simulink model "tether_dynamics"  (R2023a)
settings: Solver=ode5  StartTime=0.0  StopTime=30  FixedStep=0.0001  RelTol=1e-2
undefined symbols (not defined in the file): ext, ics, P0, P1, P10, P2, P3, P4, P5, P6, P7, P8, P9
settings Model: Creator=Dizzy  LastModifiedBy=dmmavani
settings OptimizationCC: DefaultParameterBehavior=Inlined  EnhancedBackFolding=on  PassReuseOutputArgsAs=Individual arguments  ZeroExternalMemoryAtStartup=off  ZeroInternalMemoryAtStartup=off  OptimizeBlockOrder=speed  DifferentSizesBufferReuse=on  OptimizationCustomize=off  EfficientTunableParamExpr=on
settings DebuggingCC: ParameterTunabilityLossMsg=error
settings SFSimCC: MATLABDynamicMemAlloc=off
settings RTWCC: Description=Embedded Coder  SystemTargetFile=ert.tlc  TemplateMakefile=ert_default_tmf
settings CodeAppCC: ForceParamTrailComments=on  IgnoreCustomStorageClasses=off  OperatorAnnotations=on  SimulinkDataObjDesc=on  SFDataObjDesc=on  InsertBlockDesc=on
settings ERTTargetCC: TargetLangStandard=C99 (ISO)  GenerateSampleERTMain=on  InlinedParameterPlacement=NonHierarchical  ERTCustomFileTemplate=example_file_process.tlc

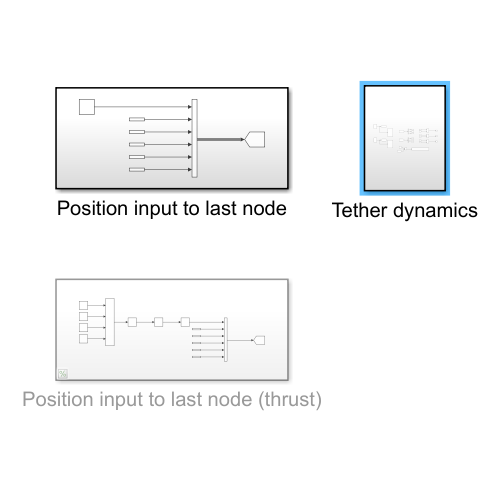
[thumbnail: Simulink's stored preview of the top-level diagram]
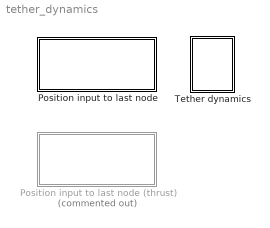
== system tether_dynamics ==
  Position input to last node : Subsystem
  Position input to last node (thrust) : Subsystem  Commented=on
  Tether dynamics : Subsystem

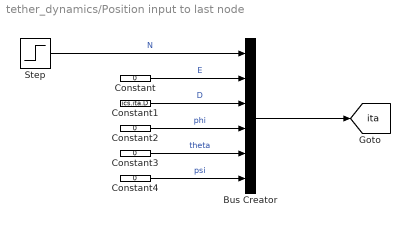
== system tether_dynamics/Position input to last node ==
  Bus Creator : BusCreator  Inputs=6  OutDataTypeStr=Bus: ita
  Constant{,2..4} (4 alike) : Constant  Value=0
  Constant1 : Constant  Value=ics.ita.D
  Step : Step  Time=0  SampleTime=0
  tag scope: ita=global
  wires:
  Constant1/1 -> Bus Creator/3  "D"
  Constant3/1 -> Bus Creator/5  "theta"
  Constant/1 -> Bus Creator/2  "E"
  Bus Creator/1 -> [ita]
  Constant2/1 -> Bus Creator/4  "phi"
  Constant4/1 -> Bus Creator/6  "psi"
  Step/1 -> Bus Creator/1  "N"

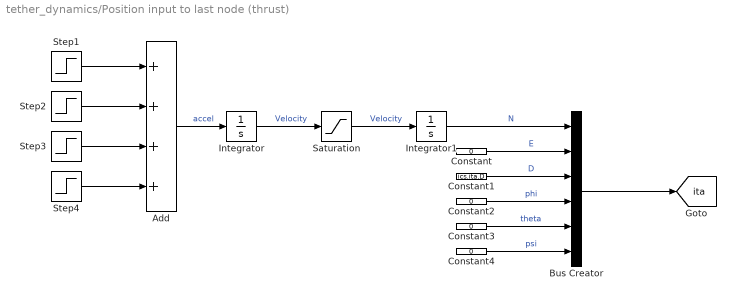
== system tether_dynamics/Position input to last node (thrust) ==
  Add : Sum  Inputs=++++
  Bus Creator : BusCreator  Inputs=6  OutDataTypeStr=Bus: ita
  Constant{,2..4} (4 alike) : Constant  Value=0
  Constant1 : Constant  Value=ics.ita.D
  Integrator : Integrator
  Integrator1 : Integrator
  Saturation : Saturate  UpperLimit=0.7  LowerLimit=0
  Step1 : Step  After=0.1  SampleTime=0
  Step2 : Step  Time=5  Before=0.1  After=0  SampleTime=0
  Step3 : Step  Time=10  After=-0.1  SampleTime=0
  Step4 : Step  Time=14  Before=-0.1  After=0  SampleTime=0
  tag scope: ita=global
  wires:
  Constant4/1 -> Bus Creator/6  "psi"
  Constant2/1 -> Bus Creator/4  "phi"
  Bus Creator/1 -> [ita]
  Constant/1 -> Bus Creator/2  "E"
  Constant3/1 -> Bus Creator/5  "theta"
  Constant1/1 -> Bus Creator/3  "D"
  Step2/1 -> Add/2
  Add/1 -> Integrator/1  "accel"
  Step1/1 -> Add/1
  Step3/1 -> Add/3
  Step4/1 -> Add/4
  Integrator/1 -> Saturation/1  "Velocity"
  Integrator1/1 -> Bus Creator/1  "N"
  Saturation/1 -> Integrator1/1  "Velocity"

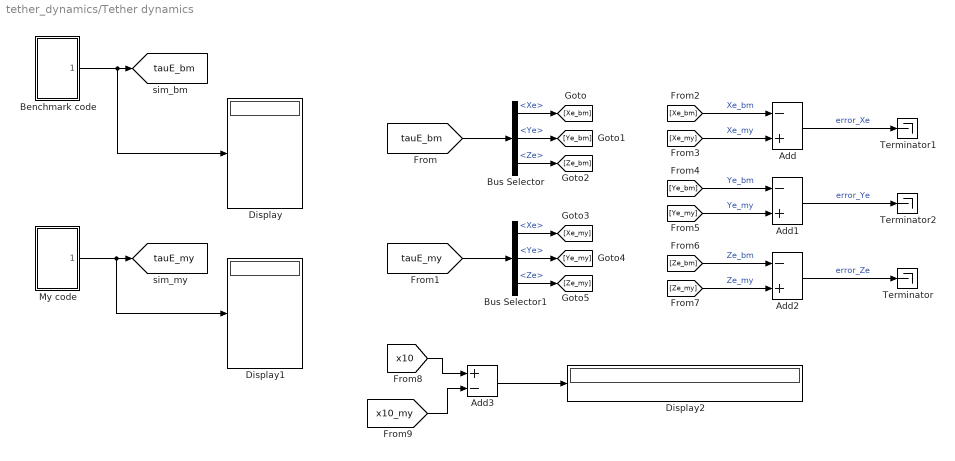
== system tether_dynamics/Tether dynamics ==
  Add : Sum  Inputs=-+
  Add1 : Sum  Inputs=-+
  Add2 : Sum  Inputs=-+
  Add3 : Sum  Inputs=+-
  Benchmark code : Subsystem
  Bus Selector : BusSelector  OutputSignals=Xe,Ye,Ze
  Bus Selector1 : BusSelector  OutputSignals=Xe,Ye,Ze
  Display : Display
  Display1 : Display
  Display2 : Display
  My code : Subsystem
  Terminator : Terminator
  Terminator1 : Terminator
  Terminator2 : Terminator
  tag scope: tauE_bm=global, tauE_my=global
  wires:
  Benchmark code/1(tauExt) -> Display/1, [tauE_bm]
  My code/1(tauExt) -> Display1/1, [tauE_my]
  [Xe_bm] -> Add/1  "Xe_bm"
  Bus Selector1/3 -> [Ze_my]  "<Ze>"
  Bus Selector/3 -> [Ze_bm]  "<Ze>"
  [tauE_my] -> Bus Selector1/1
  Bus Selector1/1 -> [Xe_my]  "<Xe>"
  [Xe_my] -> Add/2  "Xe_my"
  Add2/1 -> Terminator/1  "error_Ze"
  [Ye_bm] -> Add1/1  "Ye_bm"
  Add/1 -> Terminator1/1  "error_Xe"
  [Ze_bm] -> Add2/1  "Ze_bm"
  Bus Selector/1 -> [Xe_bm]  "<Xe>"
  [Ze_my] -> Add2/2  "Ze_my"
  Bus Selector1/2 -> [Ye_my]  "<Ye>"
  Bus Selector/2 -> [Ye_bm]  "<Ye>"
  [Ye_my] -> Add1/2  "Ye_my"
  [tauE_bm] -> Bus Selector/1
  Add1/1 -> Terminator2/1  "error_Ye"
  [x10] -> Add3/1
  [x10_my] -> Add3/2
  Add3/1 -> Display2/1

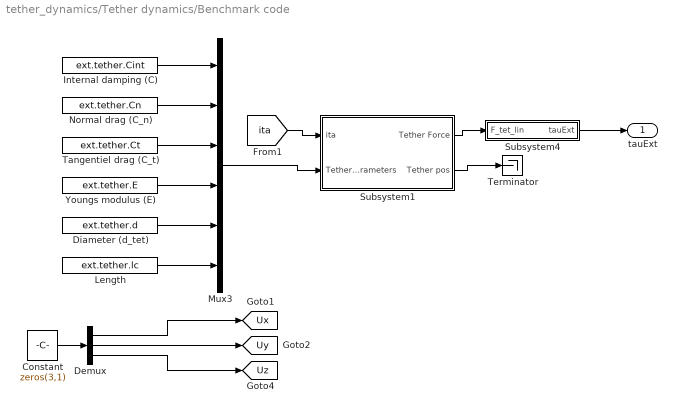
== system tether_dynamics/Tether dynamics/Benchmark code ==
  Constant : Constant  Value=zeros(3,1)
  Demux : Demux  Outputs=3
  Diameter (d_tet) : Constant  Value=ext.tether.d
  Internal damping (C) : Constant  Value=ext.tether.Cint
  Length : Constant  Value=ext.tether.lc
  Mux3 : Mux  Inputs=6
  Normal drag (C_n) : Constant  Value=ext.tether.Cn
  Subsystem1 : Subsystem
  Subsystem4 : Subsystem
  Tangentiel drag (C_t) : Constant  Value=ext.tether.Ct
  Terminator : Terminator
  Youngs modulus (E) : Constant  Value=ext.tether.E
  tauExt : Outport  OutDataTypeStr=Bus: tauExt
  tag scope: Ux=global, Uy=global, Uz=global
  wires:
  [ita] -> Subsystem1/1(ita)
  Demux/2 -> [Uy]
  Subsystem1/1(Tether Force) -> Subsystem4/1(F_tet_lin)
  Demux/3 -> [Uz]
  Constant/1 -> Demux/1
  Normal drag (C_n)/1 -> Mux3/2
  Subsystem1/2(Tether pos) -> Terminator/1
  Length/1 -> Mux3/6
  Subsystem4/1(tauExt) -> tauExt/1
  Demux/1 -> [Ux]
  Internal damping (C)/1 -> Mux3/1
  Tangentiel drag (C_t)/1 -> Mux3/3
  Diameter (d_tet)/1 -> Mux3/5
  Youngs modulus (E)/1 -> Mux3/4
  Mux3/1 -> Subsystem1/2(Tether_Parameters)

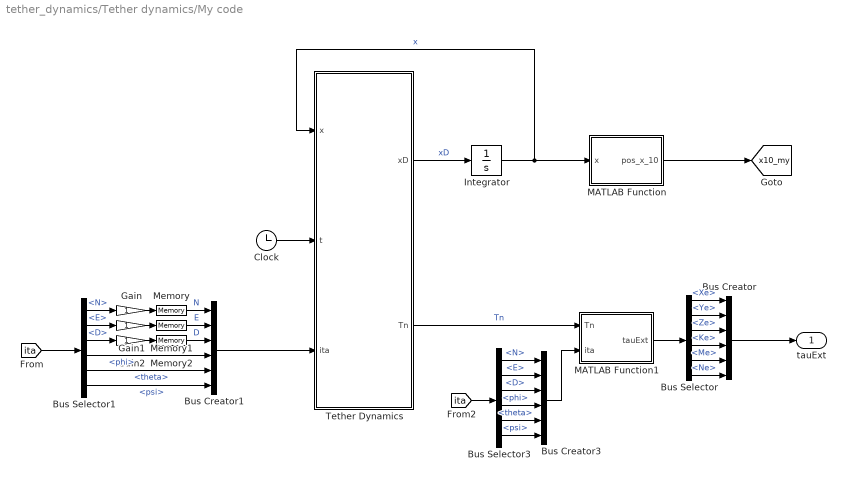
== system tether_dynamics/Tether dynamics/My code ==
  Bus Creator : BusCreator  Inputs=6  OutDataTypeStr=Bus: tauExt
  Bus Creator1 : BusCreator  Inputs=6  OutDataTypeStr=Bus: ita
  Bus Creator3 : BusCreator  Inputs=6  OutDataTypeStr=Bus: ita
  Bus Selector : BusSelector  OutputSignals=Xe,Ye,Ze,Ke,Me,Ne
  Bus Selector1 : BusSelector  OutputSignals=N,E,D,phi,theta,psi
  Bus Selector3 : BusSelector  OutputSignals=N,E,D,phi,theta,psi
  Clock : Clock
  Gain : Gain
  Gain1 : Gain
  Gain2 : Gain
  Integrator : Integrator  InitialCondition=ics.tether.xstate
  MATLAB Function : MATLAB Function  TreatAsAtomicUnit=on
  MATLAB Function1 : MATLAB Function  TreatAsAtomicUnit=on
  Memory : Memory  InitialCondition=ics.ita.N
  Memory1 : Memory  InitialCondition=ics.ita.E
  Memory2 : Memory  InitialCondition=ics.ita.D
  Tether Dynamics : MATLAB Function  TreatAsAtomicUnit=on
  tauExt : Outport  OutDataTypeStr=Bus: tauExt
  tag scope: x10_my=global
  wires:
  Bus Creator1/1 -> Tether Dynamics/3(ita)
  Bus Selector1/4 -> Bus Creator1/4  "<phi>"
  Tether Dynamics/1(xD) -> Integrator/1  "xD"
  Bus Selector3/5 -> Bus Creator3/5  "<theta>"
  Bus Selector/3 -> Bus Creator/3  "<Ze>"
  Bus Selector3/3 -> Bus Creator3/3  "<D>"
  Bus Selector1/2 -> Gain1/1  "<E>"
  Integrator/1 -> Tether Dynamics/1(x), MATLAB Function/1(x)  "x"
  Memory2/1 -> Bus Creator1/3  "D"
  Bus Selector/5 -> Bus Creator/5  "<Me>"
  Bus Creator3/1 -> MATLAB Function1/2(ita)
  Bus Selector/4 -> Bus Creator/4  "<Ke>"
  Bus Selector1/1 -> Gain/1  "<N>"
  Gain/1 -> Memory/1
  Memory/1 -> Bus Creator1/1  "N"
  Bus Selector3/6 -> Bus Creator3/6  "<psi>"
  MATLAB Function1/1(tauExt) -> Bus Selector/1
  Bus Selector3/1 -> Bus Creator3/1  "<N>"
  Bus Selector/2 -> Bus Creator/2  "<Ye>"
  Bus Selector3/2 -> Bus Creator3/2  "<E>"
  Bus Selector/6 -> Bus Creator/6  "<Ne>"
  Bus Selector3/4 -> Bus Creator3/4  "<phi>"
  Bus Selector1/3 -> Gain2/1  "<D>"
  Bus Selector/1 -> Bus Creator/1  "<Xe>"
  Tether Dynamics/2(Tn) -> MATLAB Function1/1(Tn)  "Tn"
  [ita] -> Bus Selector3/1
  Clock/1 -> Tether Dynamics/2(t)
  Bus Selector1/5 -> Bus Creator1/5  "<theta>"
  [ita] -> Bus Selector1/1
  Bus Creator/1 -> tauExt/1
  Bus Selector1/6 -> Bus Creator1/6  "<psi>"
  Gain2/1 -> Memory2/1
  Gain1/1 -> Memory1/1
  Memory1/1 -> Bus Creator1/2  "E"
  MATLAB Function/1(pos_x_10) -> [x10_my]

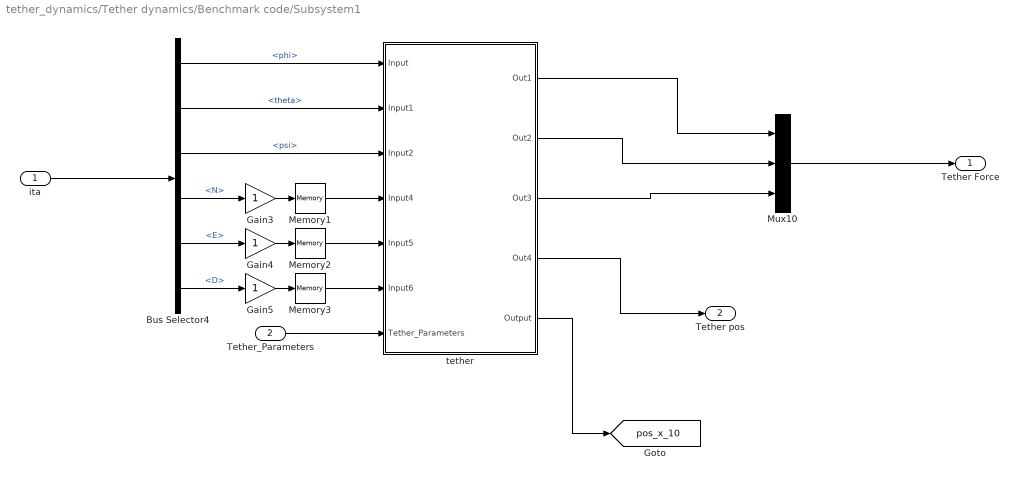
== system tether_dynamics/Tether dynamics/Benchmark code/Subsystem1 ==
  ita : Inport  OutDataTypeStr=Bus: ita
  Tether_Parameters : Inport  Port=2
  Bus Selector4 : BusSelector  OutputSignals=phi,theta,psi,N,E,D
  Gain3 : Gain
  Gain4 : Gain
  Gain5 : Gain
  Memory1 : Memory  InitialCondition=P10(1)
  Memory2 : Memory  InitialCondition=P10(2)
  Memory3 : Memory  InitialCondition=P10(3)
  Mux10 : Mux  Inputs=3
  tether : Subsystem
  Tether Force : Outport
  Tether pos : Outport  Port=2
  tag scope: pos_x_10=global
  wires:
  Memory3/1 -> tether/6(Input6)
  Memory2/1 -> tether/5(Input5)
  Memory1/1 -> tether/4(Input4)
  Bus Selector4/1 -> tether/1(Input)  "<phi>"
  Bus Selector4/2 -> tether/2(Input1)  "<theta>"
  Bus Selector4/3 -> tether/3(Input2)  "<psi>"
  Tether_Parameters/1 -> tether/7(Tether_Parameters)
  Gain3/1 -> Memory1/1
  Gain4/1 -> Memory2/1
  Gain5/1 -> Memory3/1
  tether/1(Out1) -> Mux10/1
  tether/2(Out2) -> Mux10/2
  tether/3(Out3) -> Mux10/3
  Mux10/1 -> Tether Force/1
  tether/4(Out4) -> Tether pos/1
  Bus Selector4/4 -> Gain3/1  "<N>"
  Bus Selector4/5 -> Gain4/1  "<E>"
  Bus Selector4/6 -> Gain5/1  "<D>"
  ita/1 -> Bus Selector4/1
  tether/5(Output) -> [pos_x_10]

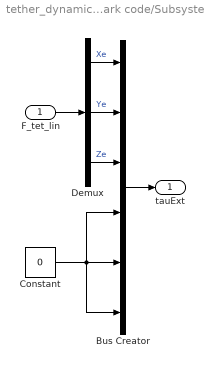
== system tether_dynamics/Tether dynamics/Benchmark code/Subsystem4 ==
  F_tet_lin : Inport
  Bus Creator : BusCreator  Inputs=6  OutDataTypeStr=Bus: tauExt
      settings: InheritFromInputs=off
  Constant : Constant  Value=0
  Demux : Demux  Outputs=3
  tauExt : Outport  OutDataTypeStr=Bus: tauExt
  wires:
  Constant/1 -> Bus Creator/6, Bus Creator/4, Bus Creator/5
  Bus Creator/1 -> tauExt/1
  Demux/1 -> Bus Creator/1  "Xe"
  Demux/2 -> Bus Creator/2  "Ye"
  Demux/3 -> Bus Creator/3  "Ze"
  F_tet_lin/1 -> Demux/1

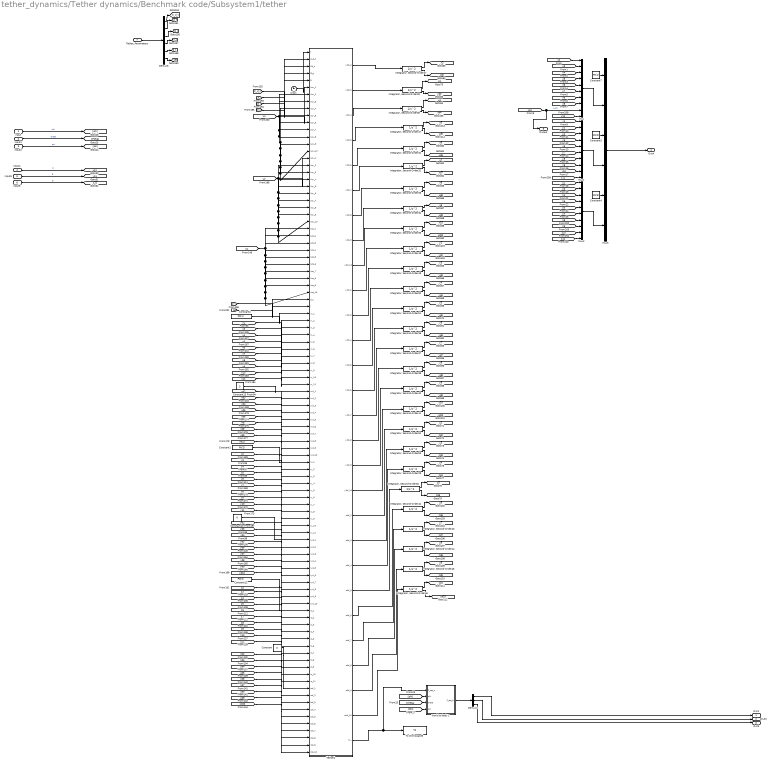
== system tether_dynamics/Tether dynamics/Benchmark code/Subsystem1/tether ==
  Input : Inport
  Input1 : Inport  Port=2
  Input2 : Inport  Port=3
  Input4 : Inport  Port=4
  Input5 : Inport  Port=5
  Input6 : Inport  Port=6
  Tether_Parameters : Inport  Port=7
  Clock : Clock
  Constant : Constant  Value=0
  Constant1 : Constant  Value=P0(2)
  Constant10 : Constant  Value=0
  Constant12 : Constant  Value=P0(3)
  Constant13 : Constant  Value=0
  Constant2 : Constant  Value=P0(1)
  Constant3 : Constant  Value=P0(2)
  Constant4 : Constant  Value=P0(3)
  Constant7 : Constant  Value=P0(1)
  Demux4 : Demux  Outputs=3
  Demux6 : Demux  Outputs=6
  "Integrator, Second-Order27" : SecondOrderIntegrator  ICX=P1(1)
  "Integrator, Second-Order28" : SecondOrderIntegrator  ICX=P2(1)
  "Integrator, Second-Order29" : SecondOrderIntegrator  ICX=P3(3)
  "Integrator, Second-Order30" : SecondOrderIntegrator  ICX=P4(3)
  "Integrator, Second-Order31" : SecondOrderIntegrator  ICX=P5(1)
  "Integrator, Second-Order32" : SecondOrderIntegrator  ICX=P6(1)
  "Integrator, Second-Order33" : SecondOrderIntegrator  ICX=P7(1)
  "Integrator, Second-Order34" : SecondOrderIntegrator  ICX=P8(1)  UpperLimitX=100  LowerLimitX=-100  UpperLimitDXDT=10  LowerLimitDXDT=-10
  "Integrator, Second-Order35" : SecondOrderIntegrator  ICX=P9(1)
  "Integrator, Second-Order36" : SecondOrderIntegrator  ICX=P5(2)
  "Integrator, Second-Order37" : SecondOrderIntegrator  ICX=P6(2)
  "Integrator, Second-Order38" : SecondOrderIntegrator  ICX=P7(2)
  "Integrator, Second-Order39" : SecondOrderIntegrator  ICX=P3(1)
  "Integrator, Second-Order40" : SecondOrderIntegrator  ICX=P8(2)
  "Integrator, Second-Order41" : SecondOrderIntegrator  ICX=P9(2)
  "Integrator, Second-Order42" : SecondOrderIntegrator  ICX=P5(3)
  "Integrator, Second-Order43" : SecondOrderIntegrator  ICX=P6(3)
  "Integrator, Second-Order44" : SecondOrderIntegrator  ICX=P7(3)
  "Integrator, Second-Order45" : SecondOrderIntegrator  ICX=P8(3)
  "Integrator, Second-Order46" : SecondOrderIntegrator  ICX=P9(3)
  "Integrator, Second-Order47" : SecondOrderIntegrator  ICX=P4(1)
  "Integrator, Second-Order48" : SecondOrderIntegrator  ICX=P1(2)
  "Integrator, Second-Order49" : SecondOrderIntegrator  ICX=P2(2)
  "Integrator, Second-Order50" : SecondOrderIntegrator  ICX=P3(2)
  "Integrator, Second-Order51" : SecondOrderIntegrator  ICX=P4(2)
  "Integrator, Second-Order52" : SecondOrderIntegrator  ICX=P1(3)
  "Integrator, Second-Order53" : SecondOrderIntegrator  ICX=P2(3)
  Mux : Mux  Inputs=10
  Mux1 : Mux  Inputs=10
  Mux2 : Mux  Inputs=10
  Mux3 : Mux  Inputs=6
  Tether2 : MATLAB Function  TreatAsAtomicUnit=on
  To Workspace3 : ToWorkspace  VariableName=T2  SaveFormat=Timeseries  SampleTime=-1
  World to body 1 : MATLAB Function  TreatAsAtomicUnit=on
  Out1 : Outport
  Out2 : Outport  Port=2
  Out3 : Outport  Port=3
  Out4 : Outport  Port=4
  Output : Outport  Port=5
  tag scope: C_d_t=global, Cd_t=global, Ct_t=global, Em_t=global, I_tet=global, d_t=global, x10=global, x11=global, x2=global, x3=global, x4=global, x5=global, x6=global, x7=global, x8=global, x9=global, xd10=global, xd2=global, xd3=global, xd4=global, xd5=global, xd6=global, xd7=global, xd8=global, xd9=global, y10=global, y11=global, y2=global, y3=global, y4=global, y5=global, y6=global, y7=global, y8=global, y9=global, yd10=global, yd2=global, yd3=global, yd4=global, yd5=global, yd6=global, yd7=global, yd8=global, yd9=global, z10=global, z11=global, z2=global, z3=global, z4=global, z5=global, z6=global, z7=global, z8=global, z9=global, zd10=global, zd2=global, zd3=global, zd4=global, zd5=global, zd6=global, zd7=global, zd8=global, zd9=global
  wires:
  Input/1 -> [phi]  "phi"
  Input1/1 -> [theta]  "theta"
  Input2/1 -> [psi]  "psi"
  Input4/1 -> [x11]  "N"
  Input5/1 -> [y11]  "E"
  Input6/1 -> [z11]  "D"
  "Integrator, Second-Order46"/1 -> [z10]
  "Integrator, Second-Order52"/1 -> [z2]
  [zd7] -> Tether2/97(rzd_7)
  "Integrator, Second-Order28"/2 -> [xd3]
  "Integrator, Second-Order36"/1 -> [y6]
  "Integrator, Second-Order32"/1 -> [x7]
  [yd7] -> Tether2/76(ryd_7)
  [zd3] -> Tether2/93(rzd_3)
  Constant12/1 -> Tether2/80(rz_1)
  "Integrator, Second-Order29"/2 -> [zd4]
  "Integrator, Second-Order29"/1 -> [z4]
  "Integrator, Second-Order35"/2 -> [xd10]
  [y5] -> Tether2/63(ry_5)
  "Integrator, Second-Order52"/2 -> [zd2]
  [z8] -> Tether2/87(rz_8)
  "Integrator, Second-Order50"/1 -> [y4]
  [y6] -> Tether2/64(ry_6)
  [xd5] -> Tether2/53(rxd_5)
  "Integrator, Second-Order50"/2 -> [yd4]
  "Integrator, Second-Order53"/1 -> [z3]
  [zd5] -> Tether2/95(rzd_5)
  [zd10] -> Tether2/100(rzd_10)
  [xd9] -> Tether2/57(rxd_9)
  [zd6] -> Tether2/96(rzd_6)
  [yd3] -> Tether2/72(ryd_3)
  "Integrator, Second-Order41"/2 -> [yd10]
  [z9] -> Tether2/88(rz_9)
  "Integrator, Second-Order38"/1 -> [y8]
  "Integrator, Second-Order31"/2 -> [xd6]
  "Integrator, Second-Order33"/2 -> [xd8]
  [yd8] -> Tether2/77(ryd_8)
  "Integrator, Second-Order41"/1 -> [y10]
  "Integrator, Second-Order30"/1 -> [z5]
  Constant1/1 -> Tether2/59(ry_1)
  [y9] -> Tether2/67(ry_9)
  "Integrator, Second-Order46"/2 -> [zd10]
  [yd10] -> Tether2/79(ryd_10)
  [z4] -> Tether2/83(rz_4)
  [y10] -> Tether2/68(ry_10)
  "Integrator, Second-Order48"/1 -> [y2]
  "Integrator, Second-Order45"/2 -> [zd9]
  [zd4] -> Tether2/94(rzd_4)
  [z11] -> Tether2/90(rz_11)
  "Integrator, Second-Order47"/2 -> [xd5]
  [y4] -> Tether2/62(ry_4)
  "Integrator, Second-Order31"/1 -> [x6]
  [z3] -> Tether2/82(rz_3)
  [xd4] -> Tether2/52(rxd_4)
  "Integrator, Second-Order37"/2 -> [yd7]
  [x7] -> Tether2/44(rx_7)
  [zd9] -> Tether2/99(rzd_9)
  [x3] -> Tether2/40(rx_3)
  [yd5] -> Tether2/74(ryd_5)
  "Integrator, Second-Order44"/2 -> [zd8]
  "Integrator, Second-Order40"/1 -> [y9]
  "Integrator, Second-Order27"/1 -> [x2]
  "Integrator, Second-Order48"/2 -> [yd2]
  [yd2] -> Tether2/71(ryd_2)
  "Integrator, Second-Order51"/2 -> [yd5]
  "Integrator, Second-Order36"/2 -> [yd6]
  "Integrator, Second-Order47"/1 -> [x5]
  "Integrator, Second-Order49"/1 -> [y3]
  "Integrator, Second-Order32"/2 -> [xd7]
  [x4] -> Tether2/41(rx_4)
  "Integrator, Second-Order45"/1 -> [z9]
  [xd8] -> Tether2/56(rxd_8)
  "Integrator, Second-Order37"/1 -> [y7]
  [z6] -> Tether2/85(rz_6)
  "Integrator, Second-Order40"/2 -> [yd9]
  "Integrator, Second-Order43"/1 -> [z7]
  "Integrator, Second-Order51"/1 -> [y5]
  Constant2/1 -> Tether2/38(rx_1)
  "Integrator, Second-Order34"/1 -> [x9]
  "Integrator, Second-Order44"/1 -> [z8]
  "Integrator, Second-Order28"/1 -> [x3]
  [z5] -> Tether2/84(rz_5)
  "Integrator, Second-Order39"/1 -> [x4]
  [z7] -> Tether2/86(rz_7)
  [z2] -> Tether2/81(rz_2)
  [xd6] -> Tether2/54(rxd_6)
  "Integrator, Second-Order34"/2 -> [xd9]
  [yd4] -> Tether2/73(ryd_4)
  [x6] -> Tether2/43(rx_6)
  [zd8] -> Tether2/98(rzd_8)
  [x8] -> Tether2/45(rx_8)
  [xd10] -> Tether2/58(rxd_10)
  [x5] -> Tether2/42(rx_5)
  [y7] -> Tether2/65(ry_7)
  [yd6] -> Tether2/75(ryd_6)
  [zd2] -> Tether2/92(rzd_2)
  "Integrator, Second-Order35"/1 -> [x10]
  [xd3] -> Tether2/51(rxd_3)
  "Integrator, Second-Order30"/2 -> [zd5]
  [y2] -> Tether2/60(ry_2)
  "Integrator, Second-Order49"/2 -> [yd3]
  "Integrator, Second-Order27"/2 -> [xd2]
  [y11] -> Tether2/69(ry_11)
  [xd7] -> Tether2/55(rxd_7)
  [yd9] -> Tether2/78(ryd_9)
  [y8] -> Tether2/66(ry_8)
  [z10] -> Tether2/89(rz_10)
  "Integrator, Second-Order42"/2 -> [zd6]
  [x10] -> Tether2/47(rx_10)
  [x2] -> Tether2/39(rx_2)
  [Uz] -> Tether2/35(Ucz_10), Tether2/34(Ucz_9), Tether2/33(Ucz_8), Tether2/32(Ucz_7), Tether2/31(Ucz_6), Tether2/30(Ucz_5), Tether2/29(Ucz_4), Tether2/28(Ucz_3), Tether2/27(Ucz_2), Tether2/26(Ucz_1)
  [x11] -> Tether2/48(rx_11)
  "Integrator, Second-Order33"/1 -> [x8]
  "Integrator, Second-Order39"/2 -> [xd4]
  "Integrator, Second-Order38"/2 -> [yd8]
  [xd2] -> Tether2/50(rxd_2)
  "Integrator, Second-Order43"/2 -> [zd7]
  "Integrator, Second-Order53"/2 -> [zd3]
  [y3] -> Tether2/61(ry_3)
  "Integrator, Second-Order42"/1 -> [z6]
  [x9] -> Tether2/46(rx_9)
  [Ux] -> Tether2/15(Ucx_10), Tether2/14(Ucx_9), Tether2/13(Ucx_8), Tether2/12(Ucx_7), Tether2/11(Ucx_6), Tether2/10(Ucx_5), Tether2/9(Ucx_4), Tether2/8(Ucx_3), Tether2/7(Ucx_2), Tether2/6(Ucx_1)
  [I_tet] -> Tether2/37(l)
  [psi] -> World to body 1/4(psi)
  World to body 1/1(F_tet_b) -> Demux4/1
  [theta] -> World to body 1/3(theta)
  [phi] -> World to body 1/2(phi)
  Tether2/28(Tix) -> World to body 1/1(F_tet_w), To Workspace3/1
  Demux4/1 -> Out1/1
  Demux4/3 -> Out3/1
  Demux4/2 -> Out2/1
  [Uy] -> Tether2/25(Ucy_10), Tether2/24(Ucy_9), Tether2/23(Ucy_8), Tether2/22(Ucy_7), Tether2/21(Ucy_6), Tether2/20(Ucy_5), Tether2/19(Ucy_4), Tether2/18(Ucy_3), Tether2/17(Ucy_2), Tether2/16(Ucy_1)
  [d_t] -> Tether2/36(d_t)
  [Cd_t] -> Tether2/3(Cd_t)
  [Ct_t] -> Tether2/4(Ct_t)
  [Em_t] -> Tether2/5(E)
  Demux6/6 -> [I_tet]
  Demux6/3 -> [Ct_t]
  Tether_Parameters/1 -> Demux6/1
  Demux6/2 -> [Cd_t]
  Demux6/5 -> [d_t]
  Demux6/4 -> [Em_t]
  [C_d_t] -> Tether2/2(C_d_t)
  Demux6/1 -> [C_d_t]
  Tether2/5(xdd_6) -> "Integrator, Second-Order31"/1
  Tether2/6(xdd_7) -> "Integrator, Second-Order32"/1
  Tether2/7(xdd_8) -> "Integrator, Second-Order33"/1
  Tether2/8(xdd_9) -> "Integrator, Second-Order34"/1
  Tether2/9(xdd_10) -> "Integrator, Second-Order35"/1
  Tether2/10(ydd_2) -> "Integrator, Second-Order48"/1
  Tether2/11(ydd_3) -> "Integrator, Second-Order49"/1
  Tether2/12(ydd_4) -> "Integrator, Second-Order50"/1
  Tether2/13(ydd_5) -> "Integrator, Second-Order51"/1
  Tether2/14(ydd_6) -> "Integrator, Second-Order36"/1
  Tether2/15(ydd_7) -> "Integrator, Second-Order37"/1
  Tether2/16(ydd_8) -> "Integrator, Second-Order38"/1
  Tether2/17(ydd_9) -> "Integrator, Second-Order40"/1
  Tether2/18(ydd_10) -> "Integrator, Second-Order41"/1
  Tether2/19(zdd_2) -> "Integrator, Second-Order52"/1
  Tether2/20(zdd_3) -> "Integrator, Second-Order53"/1
  Tether2/21(zdd_4) -> "Integrator, Second-Order29"/1
  Tether2/22(zdd_5) -> "Integrator, Second-Order30"/1
  Tether2/23(zdd_6) -> "Integrator, Second-Order42"/1
  Tether2/24(zdd_7) -> "Integrator, Second-Order43"/1
  Tether2/25(zdd_8) -> "Integrator, Second-Order44"/1
  Tether2/26(zdd_9) -> "Integrator, Second-Order45"/1
  Tether2/27(zdd_10) -> "Integrator, Second-Order46"/1
  Tether2/1(xdd_2) -> "Integrator, Second-Order27"/1
  Tether2/2(xdd_3) -> "Integrator, Second-Order28"/1
  Tether2/3(xdd_4) -> "Integrator, Second-Order39"/1
  Tether2/4(xdd_5) -> "Integrator, Second-Order47"/1
  Constant/1 -> Tether2/91(rzd_1)
  Constant10/1 -> Tether2/70(ryd_1)
  Constant13/1 -> Tether2/49(rxd_1)
  [x2] -> Mux/1
  [x3] -> Mux/2
  [x4] -> Mux/3
  [x5] -> Mux/4
  [x6] -> Mux/5
  [x7] -> Mux/6
  [x8] -> Mux/7
  [x9] -> Mux/8
  [x10] -> Output/1, Mux/9  "x_10"
  [y9] -> Mux1/8
  [y5] -> Mux1/4
  [y4] -> Mux1/3
  [y3] -> Mux1/2
  [y8] -> Mux1/7
  [y7] -> Mux1/6
  [y10] -> Mux1/9
  [y6] -> Mux1/5
  [y2] -> Mux1/1
  [z9] -> Mux2/8
  [z5] -> Mux2/4
  [z4] -> Mux2/3
  [z3] -> Mux2/2
  [z8] -> Mux2/7
  [z7] -> Mux2/6
  [z10] -> Mux2/9
  [z6] -> Mux2/5
  [z2] -> Mux2/1
  [x11] -> Mux/10
  [y11] -> Mux1/10
  [z11] -> Mux2/10
  Mux/1 -> Mux3/2
  Mux1/1 -> Mux3/4
  Mux2/1 -> Mux3/6
  Mux3/1 -> Out4/1
  Constant7/1 -> Mux3/1
  Constant3/1 -> Mux3/3
  Constant4/1 -> Mux3/5
  Clock/1 -> Tether2/1(t)

== matlab function tether_dynamics/Tether dynamics/My code/MATLAB Function ==
  data: x input; pos_x_10 output
function pos_x_10 = fcn(x)

pos = x(1:27);
pos_x_10 = pos(25);

== matlab function tether_dynamics/Tether dynamics/My code/Tether Dynamics ==
  data: x input; t input; ita input Bus: ita; xD output; Tn output; ext parameter
  function [xD,Tn] = pDD(x,t,ita,ext)
% Input by the user
%%%%%%%%%%%%%%%%%%%%%%%%%%%%%%%%%%%%%%%%%%%%%%%%%%%%
n = 9;         % no of nodes ---- (total nodes - 2)
%%%%%%%%%%%%%%%%%%%%%%%%%%%%%%%%%%%%%%%%%%%%%%%%%%%%
% if t == 4.5
%     a = 3;
%  end

l = ext.tether.lc;
E = ext.tether.E;
% m = ext.tether.m;
% l0 = ext.tether.init.lu;
% rho = phy.rho;
Cint = ext.tether.Cint;
Cn = ext.tether.Cn;
Ct = ext.tether.Ct;
dt = ext.tether.d;

xState = x;
xstate = reshape(xState,3,[]);
% let define state vector
    p0 = ext.tether.init.r0;      % position of first node
    pn = [ita.N,ita.E,ita.D]';     % position of last node (attached to ROV)
    pr = xstate(:,1:n);      % position of remaining nodes 
    v0 = zeros(3,1);
    vr = xstate(:,(n+1):(2*n));
    vc = zeros(3,1);
    
% Mass matrix
m = l * 4.3e-3;
ma = l * dt^2 * pi * 2.5e+1;
M = (m+ma) * ones(3,1); 

%% Internal forces
    % Tension in N-2 nodes  
        K = E * dt^2 * (1/l) * pi * (5/2);
        T = zeros(3,n);
        for i = 1:n
            if i<n
                % ab = l0/norm(pr(:,i+1) - pr(:,i));
                % if abs(1 - ab) < 1e-6
                %     ab = 1;
                % else
                %     % do nothing
                % end
                T(:,i) = K .* (pr(:,i)-pr(:,i+1)) .* ((l./(1.0e+1 *norm(pr(:,i) - pr(:,i+1))))-1);
            elseif i==n
                % bc = l0/norm(pn - pr(:,i));
                % if abs(1 - bc) < 1e-6
                %     bc = 1;
                % else
                %     % do nothing
                % end
                T(:,i) = K .* (pr(:,i) - pn) .* ((l./(1.0e+1 *norm(pr(:,i) - pn)))-1);
            end
        end
       
                T0 = K .* (p0 - pr(:,1)) .* ((l./(1.0e+1 * norm(p0 - pr(:,1))))-1);

    % Internal damping
        Pi = zeros(3,n);      % Internal Damping
        for i = 1:n
            if i==1
                Pi(:,i) = Cint .* (pr(:,i) - pr(:,i+1)) .* (1./norm(pr(:,i) - pr(:,i+1))) .* ((1.0e+1./l).*((pr(:,i)-pr(:,i+1))'*(v0 - vr(:,i)))) ;
            elseif (i>1)&&(i<n)
                Pi(:,i) = Cint .* (pr(:,i) - pr(:,i+1)) .* (1./norm(pr(:,i) - pr(:,i+1))) .* ((1.0e+1./l).*((pr(:,i)-pr(:,i+1))'*(vr(:,i-1) - vr(:,i))));
            elseif i == n
                Pi(:,i) = Cint .* (pr(:,i) - pn) .* (1./norm(pr(:,i) - pn)) .* ((1.0e+1./l).*((pr(:,i)-pn)'*(vr(:,i-1) - vr(:,i))));
            end
        end
                % P0 = Cint .* (p0 - pr(:,1)) .* (1./norm(p0 - pr(:,1))) .* ((1.0e+1./l).*((p0-pr(:,1))'*(v0)));
    
%% External forces
    % Hydrodynamic force/Damping
            % Normal and Tangential velocity component
                % Vt = zeros(3,n);
                % for i = 1:n
                %     if i<n
                %         Vt(:,i) = ((vc - vr(:,i))'* (pr(:,i)-pr(:,i+1))) * ((pr(:,i)-pr(:,i+1))./norm(pr(:,i)-pr(:,i+1))^2);
                %     elseif i==n
                %         Vt(:,i) = ((vc - vr(:,i))'* (pr(:,i) - pn)) * ((pr(:,i) - pn)./norm(pr(:,i) - pn)^2);
                %     end
                % end
        
                Vn = zeros(3,n);
                for i = 1:n
                    if i==1
                        Vn(:,i) = (vr(:,i)-vc) + ((vc - v0) .* (p0-pr(:,i)).^2 .* (1./norm(p0-pr(:,i)).^2));
                    else
                        Vn(:,i) = (vr(:,i)-vc) + ((vc - vr(:,i-1)) .* (pr(:,i-1)-pr(:,i)).^2 .* (1./norm(pr(:,i-1)-pr(:,i)).^2));
                    end
                end
            
               
            % Normal and tangential force component
                Fn = zeros(3,n);
                for i =1:n
                    if i<n
                        Fn(:,i) = 5.0e+2.*dt.*Cn.*Vn(:,i).* abs(Vn(:,i)).* norm(pr(:,1)-pr(:,i+1));
                    else
                        Fn(:,i) = 5.0e+2.*dt.*Cn.*Vn(:,i).* abs(Vn(:,i)).* norm(pr(:,i) - pn);
                    end
                end
            
                Ft = zeros(3,n);
                for i =1:n
                    if i<n
                        Ft(:,i) = 5.0e+2.*dt.*Ct.* norm(pr(:,i) - pr(:,i+1)) .* (vc - vr(:,i)) .* (pr(:,i) - pr(:,i+1)).^2 .* abs(pr(:,i)-pn).^2 .* (1./ norm(pr(:,i)-pr(:,i+1)).^4) .* abs(vc - vr(:,i));
                    else
                        Ft(:,i) = 5.0e+2.*dt.*Ct.* norm(pr(:,i) - pn) .* (vc - vr(:,i)) .* (pr(:,i) - pn).^2 .* abs(pr(:,i)-pn).^2 .* (1./ norm(pr(:,i)-pn).^4) .* abs(vc - vr(:,i)) ;
                    end
                end
        
            % Total hydrodynamic forces
                F = zeros(3,n);
                for i = 1:n
                    F(:,i) = (Fn(:,i) - Ft(:,i));
                end 
            

%% Equation of motion
    vd = zeros(3,n);
    for i=1:n
        if i==1
            vd(:,i) = -(T0 - T(:,i) + Pi(:,i) + F(:,i))./M;
        elseif i>1
            vd(:,i) = -(T(:,i-1) - T(:,i) - Pi(:,i-1)  + Pi(:,i)  + F(:,i))./M;
        end
    end
   
    xD = [reshape(vr,[],1);reshape(vd,[],1)];
    Tn = T(:,end);
   
   b = 5;

== matlab function tether_dynamics/Tether dynamics/My code/MATLAB Function1 ==
  data: Tn input; tauExt output Bus: tauExt; ita input
function tauExt = fcn(Tn,ita)

Rbn = rotbn(ita.phi,ita.theta,ita.psi);
Tbn = tbn(ita.phi,ita.theta);
y = [Rbn', zeros(3);zeros(3),Tbn']*[Tn;zeros(3,1)];

% Tether forces and moments
tauExt.Xe = y(1);
tauExt.Ye = y(2);
tauExt.Ze = y(3);
tauExt.Ke = y(4);
tauExt.Me = y(5);
tauExt.Ne = y(6);

== matlab function tether_dynamics/Tether dynamics/Benchmark code/Subsystem1/tether/Tether2 ==
  data: t input; C_d_t input; xdd_2 output; Cd_t input; Ct_t input; E input; Ucx_1 input; Ucx_2 input; Ucx_3 input; Ucx_4 input; Ucx_5 input; Ucx_6 input; Ucx_7 input; Ucx_8 input; Ucx_9 input; Ucx_10 input; Ucy_1 input; Ucy_2 input; Ucy_3 input; Ucy_4 input; Ucy_5 input; Ucy_6 input; Ucy_7 input; Ucy_8 input; Ucy_9 input; Ucy_10 input; Ucz_1 input; Ucz_2 input; Ucz_3 input; Ucz_4 input; Ucz_5 input; Ucz_6 input; Ucz_7 input; Ucz_8 input; Ucz_9 input; Ucz_10 input; d_t input; l input; rx_1 input; rx_2 input; rx_3 input; rx_4 input; rx_5 input; rx_6 input; rx_7 input; rx_8 input; rx_9 input; rx_10 input; rx_11 input; rxd_1 input; rxd_2 input; rxd_3 input; rxd_4 input; rxd_5 input; rxd_6 input; rxd_7 input; rxd_8 input; rxd_9 input; rxd_10 input; ry_1 input; ry_2 input; ry_3 input; ry_4 input; ry_5 input; ry_6 input; ry_7 input; ry_8 input; ry_9 input; ry_10 input; ry_11 input; ryd_1 input; ryd_2 input; ryd_3 input; ryd_4 input; ryd_5 input; ryd_6 input; ryd_7 input; ryd_8 input; ryd_9 input; ryd_10 input; rz_1 input; rz_2 input; rz_3 input; rz_4 input; rz_5 input; rz_6 input; rz_7 input; rz_8 input; rz_9 input; rz_10 input; rz_11 input; rzd_1 input; rzd_2 input; rzd_3 input; rzd_4 input; rzd_5 input; rzd_6 input; rzd_7 input; rzd_8 input; rzd_9 input; rzd_10 input; xdd_3 output; xdd_4 output; xdd_5 output; xdd_6 output; xdd_7 output; xdd_8 output; xdd_9 output; xdd_10 output; ydd_2 output; ydd_3 output; ydd_4 output; ydd_5 output; ydd_6 output; ydd_7 output; ydd_8 output; ydd_9 output; ydd_10 output; zdd_2 output; zdd_3 output; zdd_4 output; zdd_5 output; zdd_6 output; zdd_7 output; zdd_8 output; zdd_9 output; zdd_10 output; Tix output
function [xdd_2,xdd_3,xdd_4,xdd_5,xdd_6,xdd_7,xdd_8,xdd_9,xdd_10,ydd_2,ydd_3,ydd_4,ydd_5,ydd_6,ydd_7,ydd_8,ydd_9,ydd_10,zdd_2,zdd_3,zdd_4,zdd_5,zdd_6,zdd_7,zdd_8,zdd_9,zdd_10,Tix] = Tether(t,C_d_t,Cd_t,Ct_t,E,Ucx_1,Ucx_2,Ucx_3,Ucx_4,Ucx_5,Ucx_6,Ucx_7,Ucx_8,Ucx_9,Ucx_10,Ucy_1,Ucy_2,Ucy_3,Ucy_4,Ucy_5,Ucy_6,Ucy_7,Ucy_8,Ucy_9,Ucy_10,Ucz_1,Ucz_2,Ucz_3,Ucz_4,Ucz_5,Ucz_6,Ucz_7,Ucz_8,Ucz_9,Ucz_10,d_t,l,rx_1,rx_2,rx_3,rx_4,rx_5,rx_6,rx_7,rx_8,rx_9,rx_10,rx_11,rxd_1,rxd_2,rxd_3,rxd_4,rxd_5,rxd_6,rxd_7,rxd_8,rxd_9,rxd_10,ry_1,ry_2,ry_3,ry_4,ry_5,ry_6,ry_7,ry_8,ry_9,ry_10,ry_11,ryd_1,ryd_2,ryd_3,ryd_4,ryd_5,ryd_6,ryd_7,ryd_8,ryd_9,ryd_10,rz_1,rz_2,rz_3,rz_4,rz_5,rz_6,rz_7,rz_8,rz_9,rz_10,rz_11,rzd_1,rzd_2,rzd_3,rzd_4,rzd_5,rzd_6,rzd_7,rzd_8,rzd_9,rzd_10)
%#codegen

%    This function was generated by the Symbolic Math Toolbox version 8.6.
%    17-Mar-2022 13:31:39
%if simtime > 0.5


t2 = d_t.^2;
t3 = -Ucx_2;
t4 = -Ucx_3;
t5 = -Ucx_4;
t6 = -Ucx_5;
t7 = -Ucx_6;
t8 = -Ucx_7;
t9 = -Ucx_8;
t10 = -Ucx_9;
t11 = -Ucx_10;
t12 = -Ucy_2;
t13 = -Ucy_3;
t14 = -Ucy_4;
t15 = -Ucy_5;
t16 = -Ucy_6;
t17 = -Ucy_7;
t18 = -Ucy_8;
t19 = -Ucy_9;
t20 = -Ucy_10;
t21 = -Ucz_2;
t22 = -Ucz_3;
t23 = -Ucz_4;
t24 = -Ucz_5;
t25 = -Ucz_6;
t26 = -Ucz_7;
t27 = -Ucz_8;
t28 = -Ucz_9;
t29 = -Ucz_10;
t30 = 1.0./l;
t31 = -rx_2;
t32 = -rx_3;
t33 = -rx_4;
t34 = -rx_5;
t35 = -rx_6;
t36 = -rx_7;
t37 = -rx_8;
t38 = -rx_9;
t39 = -rx_10;
t40 = -rx_11;
t41 = -rxd_2;
t42 = -rxd_3;
t43 = -rxd_4;
t44 = -rxd_5;
t45 = -rxd_6;
t46 = -rxd_7;
t47 = -rxd_8;
t48 = -rxd_9;
t49 = -rxd_10;
t50 = -ry_2;
t51 = -ry_3;
t52 = -ry_4;
t53 = -ry_5;
t54 = -ry_6;
t55 = -ry_7;
t56 = -ry_8;
t57 = -ry_9;
t58 = -ry_10;
t59 = -ry_11;
t60 = -ryd_2;
t61 = -ryd_3;
t62 = -ryd_4;
t63 = -ryd_5;
t64 = -ryd_6;
t65 = -ryd_7;
t66 = -ryd_8;
t67 = -ryd_9;
t68 = -ryd_10;
t69 = -rz_2;
t70 = -rz_3;
t71 = -rz_4;
t72 = -rz_5;
t73 = -rz_6;
t74 = -rz_7;
t75 = -rz_8;
t76 = -rz_9;
t77 = -rz_10;
t78 = -rz_11;
t79 = -rzd_2;
t80 = -rzd_3;
t81 = -rzd_4;
t82 = -rzd_5;
t83 = -rzd_6;
t84 = -rzd_7;
t85 = -rzd_8;
t86 = -rzd_9;
t87 = -rzd_10;
t260 = l.*4.3e-3;
t88 = Ucx_2+t41;
t89 = Ucx_3+t42;
t90 = Ucx_4+t43;
t91 = Ucx_5+t44;
t92 = Ucx_6+t45;
t93 = Ucx_7+t46;
t94 = Ucx_8+t47;
t95 = Ucx_9+t48;
t96 = Ucx_10+t49;
t97 = Ucy_2+t60;
t98 = Ucy_3+t61;
t99 = Ucy_4+t62;
t100 = Ucy_5+t63;
t101 = Ucy_6+t64;
t102 = Ucy_7+t65;
t103 = Ucy_8+t66;
t104 = Ucy_9+t67;
t105 = Ucy_10+t68;
t106 = Ucz_2+t79;
t107 = Ucz_3+t80;
t108 = Ucz_4+t81;
t109 = Ucz_5+t82;
t110 = Ucz_6+t83;
t111 = Ucz_7+t84;
t112 = Ucz_8+t85;
t113 = Ucz_9+t86;
t114 = Ucz_10+t87;
t115 = rx_1+t31;
t116 = rx_2+t32;
t117 = rx_3+t33;
t118 = rx_4+t34;
t119 = rx_5+t35;
t120 = rx_6+t36;
t121 = rx_7+t37;
t122 = rx_8+t38;
t123 = rx_9+t39;
t124 = rx_10+t40;
t125 = rxd_1+t41;
t126 = rxd_2+t42;
t127 = rxd_3+t43;
t128 = rxd_4+t44;
t129 = rxd_5+t45;
t130 = rxd_6+t46;
t131 = rxd_7+t47;
t132 = rxd_8+t48;
t133 = rxd_9+t49;
t134 = ry_1+t50;
t135 = ry_2+t51;
t136 = ry_3+t52;
t137 = ry_4+t53;
t138 = ry_5+t54;
t139 = ry_6+t55;
t140 = ry_7+t56;
t141 = ry_8+t57;
t142 = ry_9+t58;
t143 = ry_10+t59;
t144 = ryd_1+t60;
t145 = ryd_2+t61;
t146 = ryd_3+t62;
t147 = ryd_4+t63;
t148 = ryd_5+t64;
t149 = ryd_6+t65;
t150 = ryd_7+t66;
t151 = ryd_8+t67;
t152 = ryd_9+t68;
t153 = rz_1+t69;
t154 = rz_2+t70;
t155 = rz_3+t71;
t156 = rz_4+t72;
t157 = rz_5+t73;
t158 = rz_6+t74;
t159 = rz_7+t75;
t160 = rz_8+t76;
t161 = rz_9+t77;
t162 = rz_10+t78;
t163 = rzd_1+t79;
t164 = rzd_2+t80;
t165 = rzd_3+t81;
t166 = rzd_4+t82;
t167 = rzd_5+t83;
t168 = rzd_6+t84;
t169 = rzd_7+t85;
t170 = rzd_8+t86;
t171 = rzd_9+t87;
t229 = l.*t2.*pi.*2.5e+1;
t172 = abs(t115);
t173 = abs(t116);
t174 = abs(t117);
t175 = abs(t118);
t176 = abs(t119);
t177 = abs(t120);
t178 = abs(t121);
t179 = abs(t122);
t180 = abs(t123);
t181 = abs(t124);
t182 = abs(t134);
t183 = abs(t135);
t184 = abs(t136);
t185 = abs(t137);
t186 = abs(t138);
t187 = abs(t139);
t188 = abs(t140);
t189 = abs(t141);
t190 = abs(t142);
t191 = abs(t143);
t192 = abs(t153);
t193 = abs(t154);
t194 = abs(t155);
t195 = abs(t156);
t196 = abs(t157);
t197 = abs(t158);
t198 = abs(t159);
t199 = abs(t160);
t200 = abs(t161);
t201 = abs(t162);
t202 = t115.^2;
t203 = t116.^2;
t204 = t117.^2;
t205 = t118.^2;
t206 = t119.^2;
t207 = t120.^2;
t208 = t121.^2;
t209 = t122.^2;
t210 = t123.^2;
t211 = t134.^2;
t212 = t135.^2;
t213 = t136.^2;
t214 = t137.^2;
t215 = t138.^2;
t216 = t139.^2;
t217 = t140.^2;
t218 = t141.^2;
t219 = t142.^2;
t220 = t153.^2;
t221 = t154.^2;
t222 = t155.^2;
t223 = t156.^2;
t224 = t157.^2;
t225 = t158.^2;
t226 = t159.^2;
t227 = t160.^2;
t228 = t161.^2;
t261 = rxd_1.*t30.*t115.*1.0e+1;
t262 = ryd_1.*t30.*t134.*1.0e+1;
t263 = rzd_1.*t30.*t153.*1.0e+1;
t264 = t229+t260;
t265 = t30.*t116.*t125.*1.0e+1;
t266 = t30.*t117.*t126.*1.0e+1;
t267 = t30.*t118.*t127.*1.0e+1;
t268 = t30.*t119.*t128.*1.0e+1;
t269 = t30.*t120.*t129.*1.0e+1;
t270 = t30.*t121.*t130.*1.0e+1;
t271 = t30.*t122.*t131.*1.0e+1;
t272 = t30.*t123.*t132.*1.0e+1;
t273 = t30.*t124.*t133.*1.0e+1;
t274 = t30.*t135.*t144.*1.0e+1;
t275 = t30.*t136.*t145.*1.0e+1;
t276 = t30.*t137.*t146.*1.0e+1;
t277 = t30.*t138.*t147.*1.0e+1;
t278 = t30.*t139.*t148.*1.0e+1;
t279 = t30.*t140.*t149.*1.0e+1;
t280 = t30.*t141.*t150.*1.0e+1;
t281 = t30.*t142.*t151.*1.0e+1;
t282 = t30.*t143.*t152.*1.0e+1;
t283 = t30.*t154.*t163.*1.0e+1;
t284 = t30.*t155.*t164.*1.0e+1;
t285 = t30.*t156.*t165.*1.0e+1;
t286 = t30.*t157.*t166.*1.0e+1;
t287 = t30.*t158.*t167.*1.0e+1;
t288 = t30.*t159.*t168.*1.0e+1;
t289 = t30.*t160.*t169.*1.0e+1;
t290 = t30.*t161.*t170.*1.0e+1;
t291 = t30.*t162.*t171.*1.0e+1;
t230 = t172.^2;
t231 = t173.^2;
t232 = t174.^2;
t233 = t175.^2;
t234 = t176.^2;
t235 = t177.^2;
t236 = t178.^2;
t237 = t179.^2;
t238 = t180.^2;
t239 = t181.^2;
t240 = t182.^2;
t241 = t183.^2;
t242 = t184.^2;
t243 = t185.^2;
t244 = t186.^2;
t245 = t187.^2;
t246 = t188.^2;
t247 = t189.^2;
t248 = t190.^2;
t249 = t191.^2;
t250 = t192.^2;
t251 = t193.^2;
t252 = t194.^2;
t253 = t195.^2;
t254 = t196.^2;
t255 = t197.^2;
t256 = t198.^2;
t257 = t199.^2;
t258 = t200.^2;
t259 = t201.^2;
t292 = 1.0./t264;
t363 = t261+t262+t263;
t415 = t265+t274+t283;
t416 = t266+t275+t284;
t417 = t267+t276+t285;
t418 = t268+t277+t286;
t419 = t269+t278+t287;
t420 = t270+t279+t288;
t421 = t271+t280+t289;
t422 = t272+t281+t290;
t423 = t273+t282+t291;
t293 = t230+t240+t250;
t294 = t231+t241+t251;
t295 = t232+t242+t252;
t296 = t233+t243+t253;
t297 = t234+t244+t254;
t298 = t235+t245+t255;
t299 = t236+t246+t256;
t300 = t237+t247+t257;
t301 = t238+t248+t258;
t302 = t239+t249+t259;
t303 = 1.0./t293;
t304 = 1.0./t294;
t306 = 1.0./t295;
t308 = 1.0./t296;
t310 = 1.0./t297;
t312 = 1.0./t298;
t314 = 1.0./t299;
t316 = 1.0./t300;
t318 = 1.0./t301;
t320 = 1.0./t302.^2;
t321 = sqrt(t294);
t322 = sqrt(t295);
t323 = sqrt(t296);
t324 = sqrt(t297);
t325 = sqrt(t298);
t326 = sqrt(t299);
t327 = sqrt(t300);
t328 = sqrt(t301);
t329 = sqrt(t302);
t330 = 1.0./sqrt(t293);
t305 = t304.^2;
t307 = t306.^2;
t309 = t308.^2;
t311 = t310.^2;
t313 = t312.^2;
t315 = t314.^2;
t317 = t316.^2;
t319 = t318.^2;
t331 = 1.0./t321;
t332 = 1.0./t322;
t333 = 1.0./t323;
t334 = 1.0./t324;
t335 = 1.0./t325;
t336 = 1.0./t326;
t337 = 1.0./t327;
t338 = 1.0./t328;
t339 = 1.0./t329;
t340 = (l.*t330)./1.0e+1;
t350 = Ucx_1.*t202.*t303;
t351 = Ucy_1.*t211.*t303;
t352 = Ucz_1.*t220.*t303;
t364 = t88.*t203.*t304;
t365 = t89.*t204.*t306;
t366 = t90.*t205.*t308;
t367 = t91.*t206.*t310;
t368 = t92.*t207.*t312;
t369 = t93.*t208.*t314;
t370 = t94.*t209.*t316;
t371 = t95.*t210.*t318;
t372 = t97.*t212.*t304;
t373 = t98.*t213.*t306;
t374 = t99.*t214.*t308;
t375 = t100.*t215.*t310;
t376 = t101.*t216.*t312;
t377 = t102.*t217.*t314;
t378 = t103.*t218.*t316;
t379 = t104.*t219.*t318;
t380 = t106.*t221.*t304;
t381 = t107.*t222.*t306;
t382 = t108.*t223.*t308;
t383 = t109.*t224.*t310;
t384 = t110.*t225.*t312;
t385 = t111.*t226.*t314;
t386 = t112.*t227.*t316;
t387 = t113.*t228.*t318;
t341 = (l.*t331)./1.0e+1;
t342 = (l.*t332)./1.0e+1;
t343 = (l.*t333)./1.0e+1;
t344 = (l.*t334)./1.0e+1;
t345 = (l.*t335)./1.0e+1;
t346 = (l.*t336)./1.0e+1;
t347 = (l.*t337)./1.0e+1;
t348 = (l.*t338)./1.0e+1;
t349 = (l.*t339)./1.0e+1;
t353 = t340-1.0;
t388 = rxd_2+t3+t350;
t389 = ryd_2+t12+t351;
t390 = rzd_2+t21+t352;
t391 = rxd_3+t4+t364;
t392 = rxd_4+t5+t365;
t393 = rxd_5+t6+t366;
t394 = rxd_6+t7+t367;
t395 = rxd_7+t8+t368;
t396 = rxd_8+t9+t369;
t397 = rxd_9+t10+t370;
t398 = rxd_10+t11+t371;
t399 = ryd_3+t13+t372;
t400 = ryd_4+t14+t373;
t401 = ryd_5+t15+t374;
t402 = ryd_6+t16+t375;
t403 = ryd_7+t17+t376;
t404 = ryd_8+t18+t377;
t405 = ryd_9+t19+t378;
t406 = ryd_10+t20+t379;
t407 = rzd_3+t22+t380;
t408 = rzd_4+t23+t381;
t409 = rzd_5+t24+t382;
t410 = rzd_6+t25+t383;
t411 = rzd_7+t26+t384;
t412 = rzd_8+t27+t385;
t413 = rzd_9+t28+t386;
t414 = rzd_10+t29+t387;
t451 = C_d_t.*t116.*t331.*t415;
t452 = C_d_t.*t117.*t332.*t416;
t453 = C_d_t.*t118.*t333.*t417;
t454 = C_d_t.*t119.*t334.*t418;
t455 = C_d_t.*t120.*t335.*t419;
t456 = C_d_t.*t121.*t336.*t420;
t457 = C_d_t.*t122.*t337.*t421;
t458 = C_d_t.*t123.*t338.*t422;
t459 = C_d_t.*t135.*t331.*t415;
t460 = C_d_t.*t136.*t332.*t416;
t461 = C_d_t.*t137.*t333.*t417;
t462 = C_d_t.*t138.*t334.*t418;
t463 = C_d_t.*t139.*t335.*t419;
t464 = C_d_t.*t140.*t336.*t420;
t465 = C_d_t.*t141.*t337.*t421;
t466 = C_d_t.*t142.*t338.*t422;
t467 = C_d_t.*t154.*t331.*t415;
t468 = C_d_t.*t155.*t332.*t416;
t469 = C_d_t.*t156.*t333.*t417;
t470 = C_d_t.*t157.*t334.*t418;
t471 = C_d_t.*t158.*t335.*t419;
t472 = C_d_t.*t159.*t336.*t420;
t473 = C_d_t.*t160.*t337.*t421;
t474 = C_d_t.*t161.*t338.*t422;
t354 = t341-1.0;
t355 = t342-1.0;
t356 = t343-1.0;
t357 = t344-1.0;
t358 = t345-1.0;
t359 = t346-1.0;
t360 = t347-1.0;
t361 = t348-1.0;
t362 = t349-1.0;
t424 = E.*t2.*t30.*t116.*t354.*pi.*(5.0./2.0);
xdd_2 = -t292.*(-t424+t451+d_t.*t321.*(Cd_t.*t388.*abs(t388)-Ct_t.*t88.*t203.*t231.*t305.*abs(t88)).*5.0e+2+C_d_t.*t115.*t330.*t363+E.*t2.*t30.*t115.*t353.*pi.*(5.0./2.0));
if nargout > 1
    t425 = E.*t2.*t30.*t117.*t355.*pi.*(5.0./2.0);
    xdd_3 = -t292.*(t424-t425-t451+t452+d_t.*t322.*(Cd_t.*t391.*abs(t391)-Ct_t.*t89.*t204.*t232.*t307.*abs(t89)).*5.0e+2);
end
if nargout > 2
    t426 = E.*t2.*t30.*t118.*t356.*pi.*(5.0./2.0);
    xdd_4 = -t292.*(t425-t426-t452+t453+d_t.*t323.*(Cd_t.*t392.*abs(t392)-Ct_t.*t90.*t205.*t233.*t309.*abs(t90)).*5.0e+2);
end
if nargout > 3
    t427 = E.*t2.*t30.*t119.*t357.*pi.*(5.0./2.0);
    xdd_5 = -t292.*(t426-t427-t453+t454+d_t.*t324.*(Cd_t.*t393.*abs(t393)-Ct_t.*t91.*t206.*t234.*t311.*abs(t91)).*5.0e+2);
end
if nargout > 4
    t428 = E.*t2.*t30.*t120.*t358.*pi.*(5.0./2.0);
    xdd_6 = -t292.*(t427-t428-t454+t455+d_t.*t325.*(Cd_t.*t394.*abs(t394)-Ct_t.*t92.*t207.*t235.*t313.*abs(t92)).*5.0e+2);
end
if nargout > 5
    t429 = E.*t2.*t30.*t121.*t359.*pi.*(5.0./2.0);
    xdd_7 = -t292.*(t428-t429-t455+t456+d_t.*t326.*(Cd_t.*t395.*abs(t395)-Ct_t.*t93.*t208.*t236.*t315.*abs(t93)).*5.0e+2);
end
if nargout > 6
    t430 = E.*t2.*t30.*t122.*t360.*pi.*(5.0./2.0);
    xdd_8 = -t292.*(t429-t430-t456+t457+d_t.*t327.*(Cd_t.*t396.*abs(t396)-Ct_t.*t94.*t209.*t237.*t317.*abs(t94)).*5.0e+2);
end
if nargout > 7
    t431 = E.*t2.*t30.*t123.*t361.*pi.*(5.0./2.0);
    xdd_9 = -t292.*(t430-t431-t457+t458+d_t.*t328.*(Cd_t.*t397.*abs(t397)-Ct_t.*t95.*t210.*t238.*t319.*abs(t95)).*5.0e+2);
end
if nargout > 8
    t432 = E.*t2.*t30.*t124.*t362.*pi.*(5.0./2.0);
    xdd_10 = -t292.*(t431-t432-t458+d_t.*t329.*(Cd_t.*t398.*abs(t398)-Ct_t.*t96.*t124.^2.*t239.*t320.*abs(t96)).*5.0e+2+C_d_t.*t124.*t339.*t423);
end
if nargout > 9
    t433 = E.*t2.*t30.*t135.*t354.*pi.*(5.0./2.0);
    ydd_2 = -t292.*(-t433+t459+d_t.*t321.*(Cd_t.*t389.*abs(t389)-Ct_t.*t97.*t212.*t241.*t305.*abs(t97)).*5.0e+2+C_d_t.*t134.*t330.*t363+E.*t2.*t30.*t134.*t353.*pi.*(5.0./2.0));
end
if nargout > 10
    t434 = E.*t2.*t30.*t136.*t355.*pi.*(5.0./2.0);
    ydd_3 = -t292.*(t433-t434-t459+t460+d_t.*t322.*(Cd_t.*t399.*abs(t399)-Ct_t.*t98.*t213.*t242.*t307.*abs(t98)).*5.0e+2);
end
if nargout > 11
    t435 = E.*t2.*t30.*t137.*t356.*pi.*(5.0./2.0);
    ydd_4 = -t292.*(t434-t435-t460+t461+d_t.*t323.*(Cd_t.*t400.*abs(t400)-Ct_t.*t99.*t214.*t243.*t309.*abs(t99)).*5.0e+2);
end
if nargout > 12
    t436 = E.*t2.*t30.*t138.*t357.*pi.*(5.0./2.0);
    ydd_5 = -t292.*(t435-t436-t461+t462+d_t.*t324.*(Cd_t.*t401.*abs(t401)-Ct_t.*t100.*t215.*t244.*t311.*abs(t100)).*5.0e+2);
end
if nargout > 13
    t437 = E.*t2.*t30.*t139.*t358.*pi.*(5.0./2.0);
    ydd_6 = -t292.*(t436-t437-t462+t463+d_t.*t325.*(Cd_t.*t402.*abs(t402)-Ct_t.*t101.*t216.*t245.*t313.*abs(t101)).*5.0e+2);
end
if nargout > 14
    t438 = E.*t2.*t30.*t140.*t359.*pi.*(5.0./2.0);
    ydd_7 = -t292.*(t437-t438-t463+t464+d_t.*t326.*(Cd_t.*t403.*abs(t403)-Ct_t.*t102.*t217.*t246.*t315.*abs(t102)).*5.0e+2);
end
if nargout > 15
    t439 = E.*t2.*t30.*t141.*t360.*pi.*(5.0./2.0);
    ydd_8 = -t292.*(t438-t439-t464+t465+d_t.*t327.*(Cd_t.*t404.*abs(t404)-Ct_t.*t103.*t218.*t247.*t317.*abs(t103)).*5.0e+2);
end
if nargout > 16
    t440 = E.*t2.*t30.*t142.*t361.*pi.*(5.0./2.0);
    ydd_9 = -t292.*(t439-t440-t465+t466+d_t.*t328.*(Cd_t.*t405.*abs(t405)-Ct_t.*t104.*t219.*t248.*t319.*abs(t104)).*5.0e+2);
end
if nargout > 17
    t441 = E.*t2.*t30.*t143.*t362.*pi.*(5.0./2.0);
    ydd_10 = -t292.*(t440-t441-t466+d_t.*t329.*(Cd_t.*t406.*abs(t406)-Ct_t.*t105.*t143.^2.*t249.*t320.*abs(t105)).*5.0e+2+C_d_t.*t143.*t339.*t423);
end
if nargout > 18
    t442 = E.*t2.*t30.*t154.*t354.*pi.*(5.0./2.0);
    zdd_2 = -t292.*(-t442+t467+d_t.*t321.*(Cd_t.*t390.*abs(t390)-Ct_t.*t106.*t221.*t251.*t305.*abs(t106)).*5.0e+2+C_d_t.*t153.*t330.*t363+E.*t2.*t30.*t153.*t353.*pi.*(5.0./2.0));
end
if nargout > 19
    t443 = E.*t2.*t30.*t155.*t355.*pi.*(5.0./2.0);
    zdd_3 = -t292.*(t442-t443-t467+t468+d_t.*t322.*(Cd_t.*t407.*abs(t407)-Ct_t.*t107.*t222.*t252.*t307.*abs(t107)).*5.0e+2);
end
if nargout > 20
    t444 = E.*t2.*t30.*t156.*t356.*pi.*(5.0./2.0);
    zdd_4 = -t292.*(t443-t444-t468+t469+d_t.*t323.*(Cd_t.*t408.*abs(t408)-Ct_t.*t108.*t223.*t253.*t309.*abs(t108)).*5.0e+2);
end
if nargout > 21
    t445 = E.*t2.*t30.*t157.*t357.*pi.*(5.0./2.0);
    zdd_5 = -t292.*(t444-t445-t469+t470+d_t.*t324.*(Cd_t.*t409.*abs(t409)-Ct_t.*t109.*t224.*t254.*t311.*abs(t109)).*5.0e+2);
end
if nargout > 22
    t446 = E.*t2.*t30.*t158.*t358.*pi.*(5.0./2.0);
    zdd_6 = -t292.*(t445-t446-t470+t471+d_t.*t325.*(Cd_t.*t410.*abs(t410)-Ct_t.*t110.*t225.*t255.*t313.*abs(t110)).*5.0e+2);
end
if nargout > 23
    t447 = E.*t2.*t30.*t159.*t359.*pi.*(5.0./2.0);
    zdd_7 = -t292.*(t446-t447-t471+t472+d_t.*t326.*(Cd_t.*t411.*abs(t411)-Ct_t.*t111.*t226.*t256.*t315.*abs(t111)).*5.0e+2);
end
if nargout > 24
    t448 = E.*t2.*t30.*t160.*t360.*pi.*(5.0./2.0);
    zdd_8 = -t292.*(t447-t448-t472+t473+d_t.*t327.*(Cd_t.*t412.*abs(t412)-Ct_t.*t112.*t227.*t257.*t317.*abs(t112)).*5.0e+2);
end
if nargout > 25
    t449 = E.*t2.*t30.*t161.*t361.*pi.*(5.0./2.0);
    zdd_9 = -t292.*(t448-t449-t473+t474+d_t.*t328.*(Cd_t.*t413.*abs(t413)-Ct_t.*t113.*t228.*t258.*t319.*abs(t113)).*5.0e+2);
end
if nargout > 26
    t450 = E.*t2.*t30.*t162.*t362.*pi.*(5.0./2.0);
    zdd_10 = -t292.*(t449-t450-t474+d_t.*t329.*(Cd_t.*t414.*abs(t414)-Ct_t.*t114.*t162.^2.*t259.*t320.*abs(t114)).*5.0e+2+C_d_t.*t162.*t339.*t423);
end
if nargout > 27
    Tix = [t432;t441;t450];
end


 a = 4;

%end

== matlab function tether_dynamics/Tether dynamics/Benchmark code/Subsystem1/tether/World to body 1 ==
  data: F_tet_w input; F_tet_b output; phi input; theta input; psi input
function F_tet_b = fcn(F_tet_w,phi,theta,psi)

J_Tinv=[                              cos(psi)*cos(theta)                              cos(theta)*sin(psi)         -sin(theta) 0         0                  0;
 cos(psi)*sin(phi)*sin(theta) - cos(phi)*sin(psi) cos(phi)*cos(psi) + sin(phi)*sin(psi)*sin(theta) cos(theta)*sin(phi) 0         0                  0;
 sin(phi)*sin(psi) + cos(phi)*cos(psi)*sin(theta) cos(phi)*sin(psi)*sin(theta) - cos(psi)*sin(phi) cos(phi)*cos(theta) 0         0                   0;
                                                0                                                0                   0 1         0         -sin(theta);
                                                0                                                0                   0 0  cos(phi) cos(theta)*sin(phi);
                                                0                                                0                   0 0 -sin(phi) cos(phi)*cos(theta)];


F_tet=J_Tinv*[F_tet_w(1) F_tet_w(2) F_tet_w(3) 0 0 0]';
F_tet_b=[F_tet(1) F_tet(2) F_tet(3)]';
